simulink library "fhfr"  (Simulink 8.1)
settings: Solver=ode1  StartTime=0.0  StopTime=Inf  FixedStep=0.001  RelTol=1e-3
PostLoadFcn:
  | , if any(exist('dsrtsu_mdlpostloadfcn', 'file') == [2, 3, 6]), try dsrtsu_mdlpostloadfcn('Execute', bdroot); catch fprintf('Error in PostLoadFcn (dsrtsu_mdlpostloadfcn) for model "%s":\n %s\n', bdroot, lasterr); end, end,
undefined symbols (not defined in the file or in its folder): KJUD_BrakeSupportDelay_ms, KJUD_DriverReactionDelay_ms, ZERO_FLOAT
libraries: dbdc x1, dsdc x1, hcu_lib x1
settings Model: DSRTSU_INTERNAL_RTI_VER=450  DSRTSU_INTERNAL_RTI_TYPE=rti1401  RTICANMMDATA=struct('GeneralSetupData',struct('modelroot','C:\Users\idiada\Desktop\HAITEC_Taiwan\trunk\AdasDragon\software\sw_development\arch\app\jud','generalsettings',struct('filesettings',struct('destfolder',struct('Name','RTICANMM_FILES','Check',1),'buildfolder',struct('Name','.','Check',1),'AbsDestfolder',struct('Name','C:\Users\idiada\Desktop\HAITEC_Taiwan\trunk\AdasDragon\software\sw_development\arch\app\jud\RTICANMM_FILES'),'AbsBuildfolder',struct('Name','C:\Users\idiada\Desktop\HAITEC_Taiwan\trunk\AdasDragon\software\sw_development\arch\app\jud'))),'options',struct('addpaths',1,'rmpaths',1,'addtrcexclusion',logical(1),'cannavigator',struct('checkmonitoring',0),'show_usrtrc',0,'use_usrtrc',0),'advanced',struct('options',[1 1 1 1 1 1 1 1 1 1 1 1 1 1 1 1 1 1 1 1 1 1 1 1 1 1 1 1 1 1 1 1 1 1 1 1 1 1 1 1 1 1 1 1 1 1 1 1 1 1 1 1 1 1 1 1 1 1 1 1 1 1 1 1 1 1 1 1 1 1 1 1 1 1 1 1 1 1 1 1 1 1 1 1 1 1 1 1 1 1 1 1 1 1 1 1 1 1 1 1]),'MPSetup',{{}},'modelname','fhfr','block','fhfr'))  DSRTSU_INTERNAL_RTIFPGA=40  Creator=idiada  LastModifiedBy=idiada

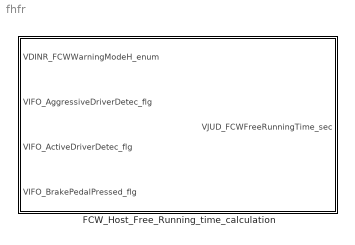
== system fhfr ==
  FCW_Host_Free_Running_time_calculation : Subsystem

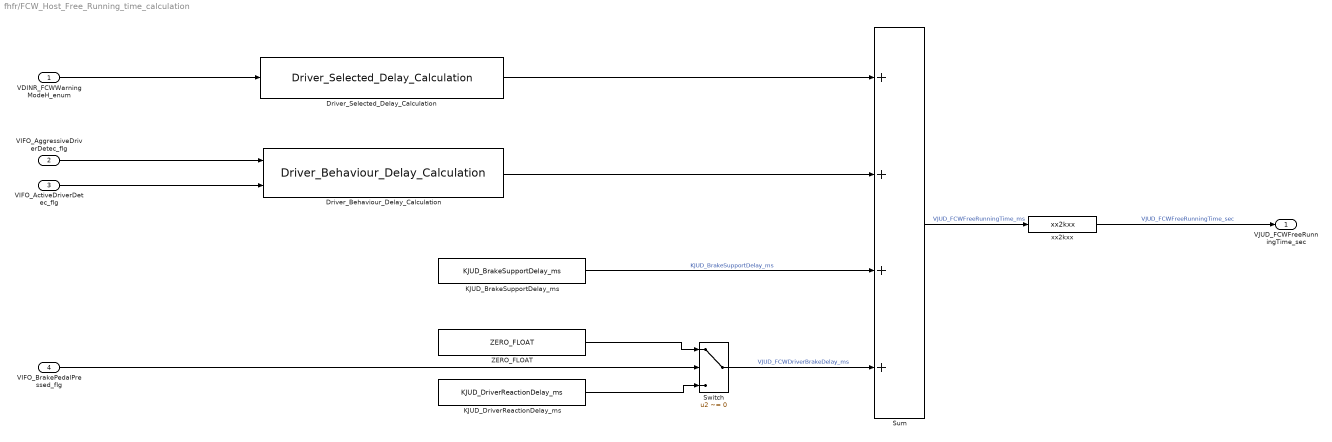
== system fhfr/FCW_Host_Free_Running_time_calculation ==
  VDINR_FCWWarningModeH_enum : Inport
  VIFO_AggressiveDriverDetec_flg : Inport  Port=2
  VIFO_ActiveDriverDetec_flg : Inport  Port=3
  VIFO_BrakePedalPressed_flg : Inport  Port=4
  Driver_Behaviour_Delay_Calculation : dbdc/Driver_Behaviour_Delay_Calculation
  Driver_Selected_Delay_Calculation : dsdc/Driver_Selected_Delay_Calculation
  KJUD_BrakeSupportDelay_ms : Constant  Value=KJUD_BrakeSupportDelay_ms
  KJUD_DriverReactionDelay_ms : Constant  Value=KJUD_DriverReactionDelay_ms
  Sum : Sum  Inputs=++++
  Switch : Switch  Criteria=u2 ~= 0
  ZERO_FLOAT : Constant  Value=ZERO_FLOAT  OutDataTypeStr=single
  xx2kxx : hcu_lib/xx2kxx
  VJUD_FCWFreeRunningTime_sec : Outport
  wires:
  xx2kxx/1 -> VJUD_FCWFreeRunningTime_sec/1  "VJUD_FCWFreeRunningTime_sec"
  VIFO_BrakePedalPressed_flg/1 -> Switch/2
  Switch/1 -> Sum/4  "VJUD_FCWDriverBrakeDelay_ms"
  ZERO_FLOAT/1 -> Switch/1
  Sum/1 -> xx2kxx/1  "VJUD_FCWFreeRunningTime_ms"
  KJUD_BrakeSupportDelay_ms/1 -> Sum/3  "KJUD_BrakeSupportDelay_ms"
  KJUD_DriverReactionDelay_ms/1 -> Switch/3
  Driver_Selected_Delay_Calculation/1 -> Sum/1
  Driver_Behaviour_Delay_Calculation/1 -> Sum/2
  VIFO_ActiveDriverDetec_flg/1 -> Driver_Behaviour_Delay_Calculation/2
  VDINR_FCWWarningModeH_enum/1 -> Driver_Selected_Delay_Calculation/1
  VIFO_AggressiveDriverDetec_flg/1 -> Driver_Behaviour_Delay_Calculation/1
